simulink model "Two_hub_motors"  (R2025b)
settings: Solver=ode4  StartTime=0.0  StopTime=10.0  FixedStep=0.001  RelTol=1e-3
model workspace (MAT data in the model file):
  T_max = 0.5
  T_min = -0.5
libraries: simulink x2, nesl_utility x1, slpidlib x1
settings Model: Creator=DELL  LastModifiedBy=DELL

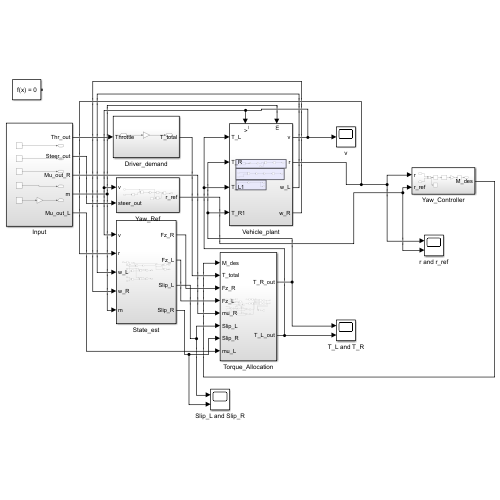
[thumbnail: Simulink's stored preview of the top-level diagram]
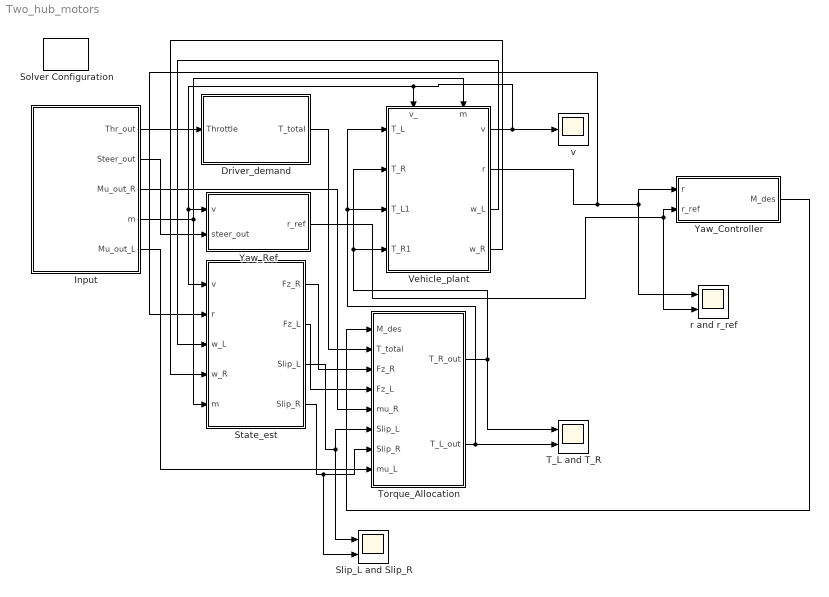
== system Two_hub_motors ==
  Driver_demand : Subsystem
  Input : Subsystem
  Slip_L and Slip_R : Scope  NumInputPorts=2
      settings: ActiveDisplayYMinimum=-0.99675909820149866  ActiveDisplayYMaximum=-0.31948839505218846  DataLoggingVariableName=ScopeData13
  Solver Configuration : nesl_utility/Solver Configuration  PhysicalDomain=network_engine_domain  SubClassName=solver  LeftPortType=input  RightPortType=generic  Tones=[]  Harmonics=[]  SimulateNoise=off  Profile=off  UseLocalSampling=off  EnableSwitchedLinearOptims=on  FrequencyDomain=off  UseCCode=off  RelTol=0.001  AbsTol=0.001  MinStep=1e-09  ToWorkspace=off  RevertToSquareIcSolve=off  NumHomotopyIterations=100  PhasorMode=off  PhasorModeNumHarmonics=1  ConsistencySolver=NEWTON_XTOL_AFTER_FTOL  IndexReductionMethod=DerivativeReplacement  DoDC=off  ResidualTolerance=1e-09  ConsistencyTolSource=GLOBAL  ConsistencyAbsTol=0.001  ConsistencyRelTol=0.001  ConsistencyTolFactor=0.001  UseLocalSolver=off  LocalSolverChoice=NE_BACKWARD_EULER_ADVANCER  ResolveIndetEquations=on  FunctionEvalNumThread=1  LocalSolverSampleTime=0.001  DoFixedCost=off  MaxNonlinIter=3  MaxModeIter=2  ComputeImpulses=off  ImpulseIterations=2  LinearAlgebra=auto  LinearAlgebraNumThread=0  EquationFormulation=NE_TIME_EF  DelaysMemoryBudget=1024  AutomaticFiltering=on  FilteringTimeConstant=0.001  PartitionStorageMethod=AS_NEEDED  PartitionMemoryBudget=1024  PartitionMethod=ROBUST  MultibodyUseLocalSolver=off  MultibodyLocalSolverChoice=ODE1  MultibodyLocalSolverSampleTime=0.001
  State_est : Subsystem
  T_L and T_R : Scope  NumInputPorts=2
      settings: ActiveDisplayYMinimum=-10.499999999999998  ActiveDisplayYMaximum=94.5  DataLoggingVariableName=ScopeData3
  Torque_Allocation : Subsystem
  Vehicle_plant : Subsystem
      settings: PortSchema="{\"entries\":[{\"content\":{\"sides\":[{\"content\":{\"connectorIds\":[\"In1\",\"In2\",\"In3\",\"In4\"]},\"type\":\"ConnectorPlacement.EquallySpacedRectSide\",\"uuid\":\"46f6a90a-06e8-4a4f-aff5-b58e133d1555\"},{\"content\":{\"connectorIds\":[\"Out1\",\"Out2\",\"Out3\",\"Out4\"],\"side\":\"RIGHT\"},\"type\":\"ConnectorPlacement.EquallySpacedRectSide\",\"uuid\":\"3acb0db9-baac-4fda-989c-d7b4b0dfc613\"},{\"content\":{\"connectorIds\":[\"In5\",\"In6\"],\"side\":\"TOP\"},\"type\":\"ConnectorPlacement.EquallySpacedRectSide\",\"uuid\":\"0c5a56e6-ec3c-426a-9dc4-4288964cc701\"}]},\"type\":\"ConnectorPlacement.EquallySpacedConnector\",\"uuid\":\"cb05e45d-f259-45e3-9f35-21bfd16cc93b\"}],\"packageUris\":[\"http://schema.mathworks.com/mf0/Connector/R2020b\"],\"version\":\"1.0\"}"
  Yaw_Controller : Subsystem
  Yaw_Ref : Subsystem
  r and r_ref : Scope  NumInputPorts=2
      settings: ActiveDisplayYMinimum=-0.10408935150215097  ActiveDisplayYMaximum=0.936804163519359
  v : Scope
      settings: ActiveDisplayYMinimum=-5.9204298341374653  ActiveDisplayYMaximum=12.566767753770838
  wires:
  Input/1(Thr_out) -> Driver_demand/1(Throttle)
  Input/2(Steer_out) -> Yaw_Ref/2(steer_out)
  Input/3(Mu_out_R) -> Torque_Allocation/5(mu_R)
  Driver_demand/1(T_total) -> Torque_Allocation/2(T_total)
  Vehicle_plant/1(v) -> v/1, State_est/1(v), Yaw_Ref/1(v), Vehicle_plant/5(v_)
  Yaw_Ref/1(r_ref) -> r and r_ref/2, Yaw_Controller/2(r_ref)
  Vehicle_plant/3(w_L) -> State_est/3(w_L)
  Vehicle_plant/4(w_R) -> State_est/4(w_R)
  Yaw_Controller/1(M_des) -> Torque_Allocation/1(M_des)
  Torque_Allocation/1(T_R_out) -> T_L and T_R/1, Vehicle_plant/2(T_R), Vehicle_plant/4(T_R1)
  Torque_Allocation/2(T_L_out) -> Vehicle_plant/1(T_L), Vehicle_plant/3(T_L1), T_L and T_R/2
  State_est/3(Slip_L) -> Torque_Allocation/6(Slip_L), Slip_L and Slip_R/1
  State_est/4(Slip_R) -> Slip_L and Slip_R/2, Torque_Allocation/7(Slip_R)
  State_est/1(Fz_R) -> Torque_Allocation/3(Fz_R)
  State_est/2(Fz_L) -> Torque_Allocation/4(Fz_L)
  Vehicle_plant/2(r) -> State_est/2(r), r and r_ref/1, Yaw_Controller/1(r)
  Input/4(m) -> Vehicle_plant/6(m), State_est/5(m)
  Input/5(Mu_out_L) -> Torque_Allocation/8(mu_L)

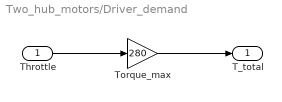
== system Two_hub_motors/Driver_demand ==
  Throttle : Inport
  Torque_max : Gain  Gain=280
  T_total : Outport
  wires:
  Throttle/1 -> Torque_max/1
  Torque_max/1 -> T_total/1

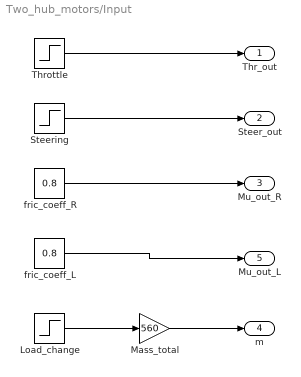
== system Two_hub_motors/Input ==
  Load_change : Step  Before=0.78  SampleTime=0
  Mass_total : Gain  Gain=560
  Steering : Step  After=0.15  SampleTime=0
  Throttle : Step  Time=0.5  After=0.6  SampleTime=0
  fric_coeff_L : Constant  Value=0.8
  fric_coeff_R : Constant  Value=0.8
  Thr_out : Outport
  Steer_out : Outport  Port=2
  Mu_out_R : Outport  Port=3
  m : Outport  Port=4
  Mu_out_L : Outport  Port=5
  wires:
  Throttle/1 -> Thr_out/1
  Steering/1 -> Steer_out/1
  fric_coeff_R/1 -> Mu_out_R/1
  fric_coeff_L/1 -> Mu_out_L/1
  Load_change/1 -> Mass_total/1
  Mass_total/1 -> m/1

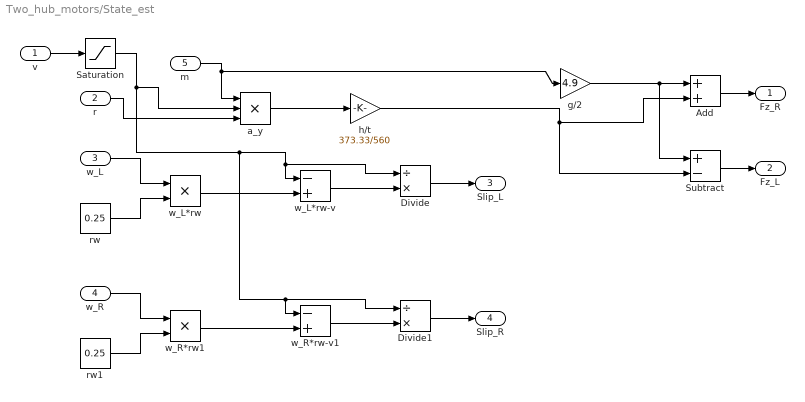
== system Two_hub_motors/State_est ==
  v : Inport
  r : Inport  Port=2
  w_L : Inport  Port=3
  w_R : Inport  Port=4
  m : Inport  Port=5
  Add : Sum
  Divide : Product  Inputs=/*
  Divide1 : Product  Inputs=/*
  Saturation : Saturate  UpperLimit=Inf  LowerLimit=0.5
  Subtract : Sum  Inputs=+-
  a_y : Product  Inputs=3
  g/2 : Gain  Gain=4.9
  h/t : Gain  Gain=373.33/560
  rw : Constant  Value=0.25
  rw1 : Constant  Value=0.25
  w_L*rw : Product
  w_L*rw-v : Sum  Inputs=-+
  w_R*rw-v1 : Sum  Inputs=-+
  w_R*rw1 : Product
  Fz_R : Outport
  Fz_L : Outport  Port=2
  Slip_L : Outport  Port=3
  Slip_R : Outport  Port=4
  wires:
  r/1 -> a_y/3
  a_y/1 -> h/t/1
  h/t/1 -> Subtract/2, Add/2
  g/2/1 -> Subtract/1, Add/1
  Add/1 -> Fz_R/1
  Subtract/1 -> Fz_L/1
  w_L/1 -> w_L*rw/1
  rw/1 -> w_L*rw/2
  w_L*rw/1 -> w_L*rw-v/2
  w_L*rw-v/1 -> Divide/2
  Divide/1 -> Slip_L/1
  rw1/1 -> w_R*rw1/2
  w_R*rw-v1/1 -> Divide1/2
  Divide1/1 -> Slip_R/1
  w_R*rw1/1 -> w_R*rw-v1/2
  w_R/1 -> w_R*rw1/1
  Saturation/1 -> a_y/2, w_L*rw-v/1, Divide/1, Divide1/1, w_R*rw-v1/1
  v/1 -> Saturation/1
  m/1 -> a_y/1, g/2/1

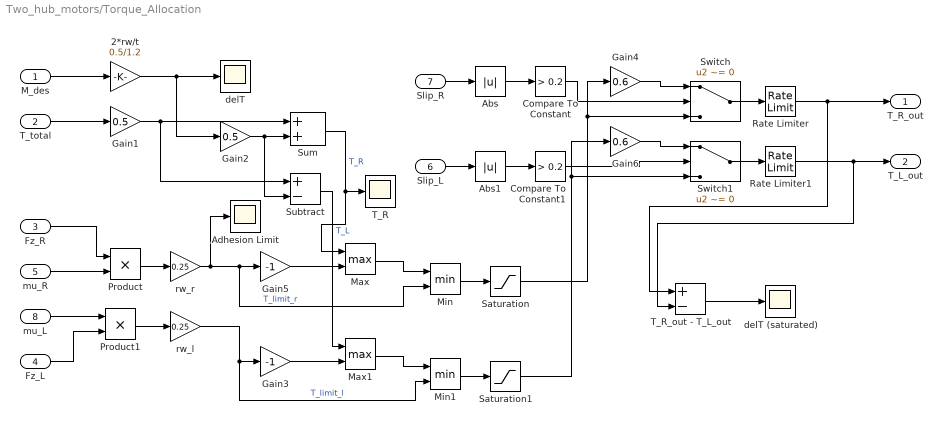
== system Two_hub_motors/Torque_Allocation ==
  M_des : Inport
  T_total : Inport  Port=2
  Fz_R : Inport  Port=3
  Fz_L : Inport  Port=4
  mu_R : Inport  Port=5
  Slip_L : Inport  Port=6
  Slip_R : Inport  Port=7
  mu_L : Inport  Port=8
  2*rw/t : Gain  Gain=0.5/1.2
  Abs : Abs  SaturateOnIntegerOverflow=off
  Abs1 : Abs  SaturateOnIntegerOverflow=off
  Adhesion Limit : Scope
      settings: ActiveDisplayYMinimum=-1  ActiveDisplayYMaximum=1  DataLoggingVariableName=ScopeData12
  Compare To Constant : simulink/Logic and Bit Operations/Compare To Constant  relop=>  const=0.2  OutDataTypeStr=boolean
  Compare To Constant1 : simulink/Logic and Bit Operations/Compare To Constant  relop=>  const=0.2  OutDataTypeStr=boolean
  Gain1 : Gain  Gain=0.5
  Gain2 : Gain  Gain=0.5
  Gain3 : Gain  Gain=-1
  Gain4 : Gain  Gain=0.6
  Gain5 : Gain  Gain=-1
  Gain6 : Gain  Gain=0.6
  Max : MinMax  Function=max  Inputs=2
  Max1 : MinMax  Function=max  Inputs=2
  Min : MinMax  Inputs=2
  Min1 : MinMax  Inputs=2
  Product : Product
  Product1 : Product
  Rate Limiter : RateLimiter  RisingSlewLimit=600  FallingSlewLimit=-600  SampleTimeMode=inherited
  Rate Limiter1 : RateLimiter  RisingSlewLimit=600  FallingSlewLimit=-600  SampleTimeMode=inherited
  Saturation : Saturate  UpperLimit=140  LowerLimit=-140
  Saturation1 : Saturate  UpperLimit=140  LowerLimit=-140
  Subtract : Sum  Inputs=+-
  Sum : Sum
  Switch : Switch  Criteria=u2 ~= 0  SaturateOnIntegerOverflow=off  InputSameDT=off
  Switch1 : Switch  Criteria=u2 ~= 0  SaturateOnIntegerOverflow=off  InputSameDT=off
  T_R : Scope
      settings: DataLoggingVariableName=ScopeData10
  T_R_out - T_L_out : Sum  Inputs=+-
  delT : Scope
      settings: ActiveDisplayYMinimum=-102.43514068264402  ActiveDisplayYMaximum=218.25745954745065  DataLoggingVariableName=ScopeData4
  delT (saturated) : Scope
      settings: ActiveDisplayYMinimum=-1  ActiveDisplayYMaximum=1  DataLoggingVariableName=ScopeData9
  rw_l : Gain  Gain=0.25
  rw_r : Gain  Gain=0.25
  T_R_out : Outport
  T_L_out : Outport  Port=2
  wires:
  M_des/1 -> 2*rw/t/1
  2*rw/t/1 -> delT/1, Gain2/1
  T_total/1 -> Gain1/1
  Gain1/1 -> Subtract/1, Sum/1
  Gain2/1 -> Subtract/2, Sum/2
  Sum/1 -> T_R/1, Max/1  "T_R"
  Fz_R/1 -> Product/1
  mu_R/1 -> Product/2
  Product/1 -> rw_r/1
  Fz_L/1 -> Product1/2
  Product1/1 -> rw_l/1
  rw_r/1 -> Adhesion Limit/1, Min/2, Gain5/1  "T_limit_r"
  Gain5/1 -> Max/2
  Max/1 -> Min/1
  Subtract/1 -> Max1/1  "T_L"
  Max1/1 -> Min1/1
  Gain3/1 -> Max1/2
  Min/1 -> Saturation/1
  Saturation/1 -> Switch/3, Gain4/1
  Min1/1 -> Saturation1/1
  Abs/1 -> Compare To Constant/1
  Abs1/1 -> Compare To Constant1/1
  Gain4/1 -> Switch/1
  Compare To Constant/1 -> Switch/2
  Slip_L/1 -> Abs1/1
  Slip_R/1 -> Abs/1
  Gain6/1 -> Switch1/1
  rw_l/1 -> Min1/2, Gain3/1  "T_limit_l"
  Compare To Constant1/1 -> Switch1/2
  Saturation1/1 -> Switch1/3, Gain6/1
  Switch/1 -> Rate Limiter/1
  Switch1/1 -> Rate Limiter1/1
  Rate Limiter/1 -> T_R_out/1, T_R_out - T_L_out/1
  Rate Limiter1/1 -> T_R_out - T_L_out/2, T_L_out/1
  T_R_out - T_L_out/1 -> delT (saturated)/1
  mu_L/1 -> Product1/1

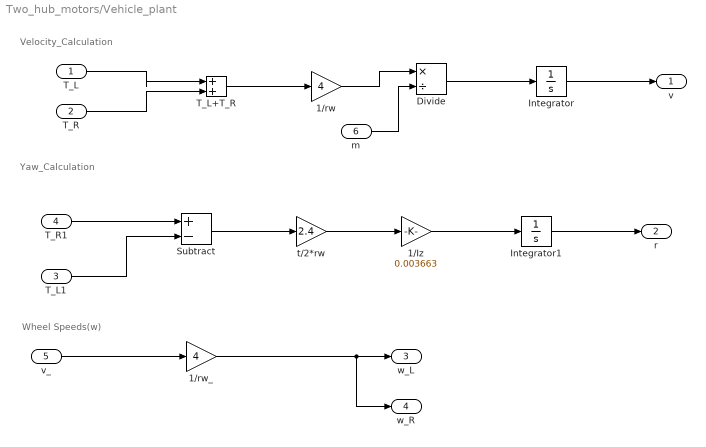
== system Two_hub_motors/Vehicle_plant ==
  note: Velocity_Calculation
  note: Yaw_Calculation
  note: Wheel Speeds(w)
  T_L : Inport
  T_R : Inport  Port=2
  T_L1 : Inport  Port=3
  T_R1 : Inport  Port=4
  v_ : Inport  Port=5
  m : Inport  Port=6
  1/Iz : Gain  Gain=0.003663
  1/rw : Gain  Gain=4
  1/rw_ : Gain  Gain=4
  Divide : Product  Inputs=*/
  Integrator : Integrator
  Integrator1 : Integrator
  Subtract : Sum  Inputs=+-
  T_L+T_R : Sum  Inputs=|++
  t/2*rw : Gain  Gain=2.4
  v : Outport  VectorParamsAs1DForOutWhenUnconnected=off
  r : Outport  Port=2  VectorParamsAs1DForOutWhenUnconnected=off
  w_L : Outport  Port=3  VectorParamsAs1DForOutWhenUnconnected=off
  w_R : Outport  Port=4  VectorParamsAs1DForOutWhenUnconnected=off
  wires:
  T_L/1 -> T_L+T_R/1
  T_R/1 -> T_L+T_R/2
  T_L+T_R/1 -> 1/rw/1
  1/rw/1 -> Divide/1
  T_L1/1 -> Subtract/2
  Subtract/1 -> t/2*rw/1
  t/2*rw/1 -> 1/Iz/1
  1/rw_/1 -> w_R/1, w_L/1
  v_/1 -> 1/rw_/1
  T_R1/1 -> Subtract/1
  Divide/1 -> Integrator/1
  Integrator/1 -> v/1
  1/Iz/1 -> Integrator1/1
  Integrator1/1 -> r/1
  m/1 -> Divide/2

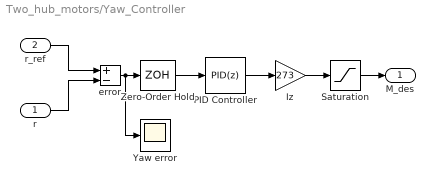
== system Two_hub_motors/Yaw_Controller ==
  r : Inport
  r_ref : Inport  Port=2
  Iz : Gain  Gain=273
  PID Controller : slpidlib/PID Controller  Controller=PID  Form=Parallel  TimeDomain=Discrete-time  UseExternalTs=off  SampleTime=0.01  IntegratorMethod=Forward Euler  FilterMethod=Forward Euler  ControllerParametersSource=internal  P=8  I=0  UseKiTs=off  D=0  UseExternalDerivativeSource=off  N=20  UseFilter=on  TunerSelectOption=Transfer Function Based (PID Tuner App)  InitialConditionSource=internal  InitialConditionForIntegrator=0  InitialConditionForFilter=0  DifferentiatorICPrevScaledInput=0  ExternalReset=none  TrackingMode=off  Kt=1  LimitOutput=on  SatLimitsSource=internal  UpperSaturationLimit=inf  LowerSaturationLimit=-inf  LinearizeAsGain=on  AntiWindupMode=clamping  Kb=1  LimitIntegrator=off  UpperIntegratorSaturationLimit=inf  LowerIntegratorSaturationLimit=-inf  POutMin=[]  POutMax=[]  IOutMin=[]  IOutMax=[]  DOutMin=[]  DOutMax=[]  NOutMin=[]  NOutMax=[]  SumOutMin=[]  SumOutMax=[]  SaturationOutMin=[]  SaturationOutMax=[]  PParamMin=[]  PParamMax=[]  IParamMin=[]  IParamMax=[]  DParamMin=[]  DParamMax=[]  NParamMin=[]  NParamMax=[]  KbParamMin=[]  KbParamMax=[]  KtParamMin=[]  KtParamMax=[]  KbOutMin=[]  KbOutMax=[]  KtOutMin=[]  KtOutMax=[]  IntegratorOutMin=[]  IntegratorOutMax=[]  FilterOutMin=[]  FilterOutMax=[]  SumI1OutMin=[]  SumI1OutMax=[]  SumI2OutMin=[]  SumI2OutMax=[]  SumI3OutMin=[]  SumI3OutMax=[]  SumI4OutMin=[]  SumI4OutMax=[]  SumDOutMin=[]  SumDOutMax=[]  DifferentiatorOutMin=[]  DifferentiatorOutMax=[]  FilterDiffOutCoefMin=[]  FilterDiffOutCoefMax=[]  ReciprocalOutMin=[]  ReciprocalOutMax=[]  SumDenOutMin=[]  SumDenOutMax=[]  SumNumOutMin=[]  SumNumOutMax=[]  DivideOutMin=[]  DivideOutMax=[]  UdiffTsProdOutMin=[]  UdiffTsProdOutMax=[]  NTsProdOutMin=[]  NTsProdOutMax=[]  UintegralTsProdOutMin=[]  UintegralTsProdOutMax=[]  UngainTsProdOutMin=[]  UngainTsProdOutMax=[]  ClampingZeroOutDataTypeStr=Inherit: Inherit via back propagation  ClampingZeroOutMin=[]  ClampingZeroOutMax=[]  FilterDenConstantOutDataTypeStr=Inherit: Inherit via back propagation  FilterDenConstantOutMin=[]  FilterDenConstantOutMax=[]  PCopyOutDataTypeStr=Inherit: Inherit via back propagation  PCopyOutMin=[]  PCopyOutMax=[]  NCopyOutDataTypeStr=Inherit: Inherit via back propagation  NCopyOutMin=[]  NCopyOutMax=[]  IntegratorContinuousStateAttributes=''  IntegratorStateMustResolveToSignalObject=off  IntegratorRTWStateStorageClass=Auto  FilterContinuousStateAttributes=''  FilterStateMustResolveToSignalObject=off  FilterRTWStateStorageClass=Auto  ParallelPVariant=InternalParameters  IdealPVariant=Disabled  IVariant=InternalParameters  DVariant=InternalParameters  IntegratorVariant=Discrete  SatVariant=Enabled  AWVariant=DiscClampingParallel  PCopyVariant=Disabled  TRVariant=Disabled  FdbkBlocksVariant=Forward  IdealPFdbkVariant=Disabled  SatFdbkVariant=Disabled  DerivativeFilterVariant=ForwardEulerFilter  NVariant=InternalParameters  NCopyVariant=Disabled  FilterICVariant=InternalICsFilter  IntegratorICVariant=InternalICs  ExternalResetVariant=Disabled  TRSumVariant=Passthrough  SumFdbkVariant=Disabled  SumVariant=Sum_PID  TsampFilterVariant=InternalTs  TsampNgainVariant=Passthrough  TsampIntegralVariant=Disabled_SignalSpec  ExternalSaturationOutDataTypeStr=Inherit: Same as second input  DerivativeSourceVariant=ErrorSignal  PreIntVariant=InternalPreInt
  Saturation : Saturate  UpperLimit=600  LowerLimit=-600
  Yaw error : Scope
      settings: ActiveDisplayYMinimum=-0.21574055215157698  ActiveDisplayYMaximum=0.050700915649022175  DataLoggingVariableName=ScopeData8
  Zero-Order Hold : ZeroOrderHold  SampleTime=0.01
  error : Sum  Inputs=+-
  M_des : Outport
  wires:
  r_ref/1 -> error/1
  r/1 -> error/2
  PID Controller/1 -> Iz/1
  Iz/1 -> Saturation/1
  Saturation/1 -> M_des/1
  error/1 -> Yaw error/1, Zero-Order Hold/1
  Zero-Order Hold/1 -> PID Controller/1

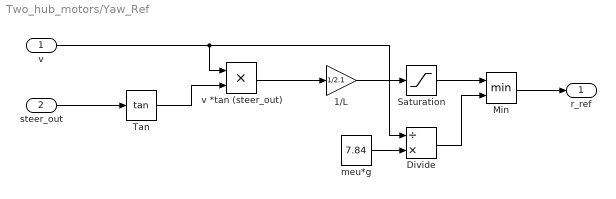
== system Two_hub_motors/Yaw_Ref ==
  v : Inport
  steer_out : Inport  Port=2
  1/L : Gain  Gain=1/2.1
  Divide : Product  Inputs=/*
  Min : MinMax  Inputs=2
  Saturation : Saturate  UpperLimit=0.6  LowerLimit=-0.6
  Tan : Trigonometry  Operator=tan
  meu*g : Constant  Value=7.84
  v *tan (steer_out) : Product
  r_ref : Outport
  wires:
  steer_out/1 -> Tan/1
  Tan/1 -> v *tan (steer_out)/2
  v/1 -> Divide/1, v *tan (steer_out)/1
  v *tan (steer_out)/1 -> 1/L/1
  1/L/1 -> Saturation/1
  meu*g/1 -> Divide/2
  Saturation/1 -> Min/1
  Divide/1 -> Min/2
  Min/1 -> r_ref/1
